simulink model "simu_receive"  (Simulink 7.6)
settings: Solver=FixedStepDiscrete  StartTime=0.0  StopTime=inf  FixedStep=0.001  RelTol=1e-3
undefined symbols (not defined in the file): serial
libraries: instrumentlib x3, simulink x1
settings Model: Creator=Liran  LastModifiedBy=Liran  BufferReuse=off
settings OptimizationCC: BlockReduction=off  OptimizeBlockIOStorage=off  BufferReuse=off  ExpressionFolding=off  LocalBlockOutputs=off

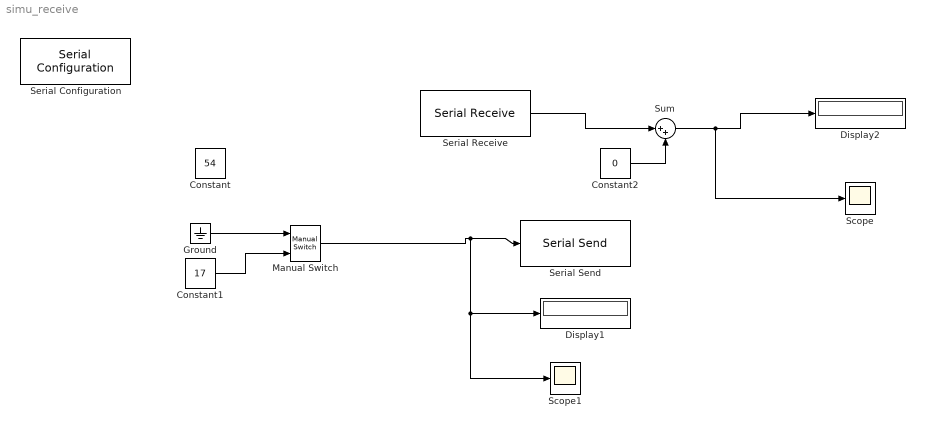
== system simu_receive ==
  Constant : Constant  Value=54  OutDataTypeStr=uint8  SampleTime=-1
  Constant1 : Constant  Value=17  OutDataTypeStr=uint8  SampleTime=-1
  Constant2 : Constant  Value=0  OutDataTypeStr=uint8  SampleTime=-1
  Display1 : Display
      settings: Format=hex (Stored Integer)
  Display2 : Display
      settings: Format=hex (Stored Integer)
  Ground : Ground
  Manual Switch : simulink/Signal Routing/Manual Switch  SystemSampleTime=-1  sw=1  action=0  varsize=off
  Scope : Scope
      settings: TimeRange=10  YMin=51.3  YMax=56.7  SaveName=output  MaxDataPoints=500000
  Scope1 : Scope
      settings: TimeRange=10  YMin=51.3  YMax=56.7  SaveName=input  MaxDataPoints=500000
  Serial Configuration : instrumentlib/Serial Configuration  Priority=-200000  DialogController=instrumentcreatedialog  DialogControllerArgs=DataTag0  ComPortMenu=COM1  ComPort=COM1  ObjConstructor=serial('COM1');  BaudRate=38400  DataBits=8  Parity=none  StopBits=1  FlowControl=none  Timeout=10  ByteOrder=LittleEndian
  Serial Receive : instrumentlib/Serial Receive  DialogController=instrumentcreatedialog  DialogControllerArgs=DataTag1  ComPortMenu=COM1  ComPort=COM1  ObjConstructor=serial('COM1');  Terminator=<none>  DataSize=1  DataType=uint8  EnableBlockingMode=on  ActionDataUnavailable=Output custom value  CustomValue=-25  SampleTime=0.001
  Serial Send : instrumentlib/Serial Send  DialogController=instrumentcreatedialog  DialogControllerArgs=DataTag2  ComPortMenu=COM1  ComPort=COM1  ObjConstructor=serial('COM1');  Terminator=<none>  EnableBlockingMode=off
  Sum : Sum  Inputs=|++
  wires:
  Manual Switch/1 -> Serial Send/1, Display1/1, Scope1/1
  Constant1/1 -> Manual Switch/2
  Sum/1 -> Display2/1, Scope/1
  Constant2/1 -> Sum/2
  Serial Receive/1 -> Sum/1
  Ground/1 -> Manual Switch/1
